simulink model "twoD_ground"  (R2022b)
settings: Solver=FixedStepAuto  StartTime=0.0  StopTime=1  FixedStep=10e-4  RelTol=1e-3
values from neighbouring files (symbols this model uses):
  bl = 0.1    [twoD.m]
  bw = 0.001    [twoD.m]
  g = 9.81    [twoD.m]
  I = m*(e^2 + n^2)/12    (= 0.001875)    [twoD.m]
  k0 = 1000    [twoD.m]
  Kf = acker(Af,Bf,Poles)    [twoD.m]
  l0 = 0.3    [twoD.m]
  m = 0.5    [twoD.m]
  Nf = rscale(Gp,Kf)    [twoD.m]
  Ng = rscale(sys,Kg)    [twoD.m]
undefined symbols (not defined in the file or in its folder): Kg
libraries: simulink x2
settings Model: Creator=phattanarat  LastModifiedBy=phattanarat

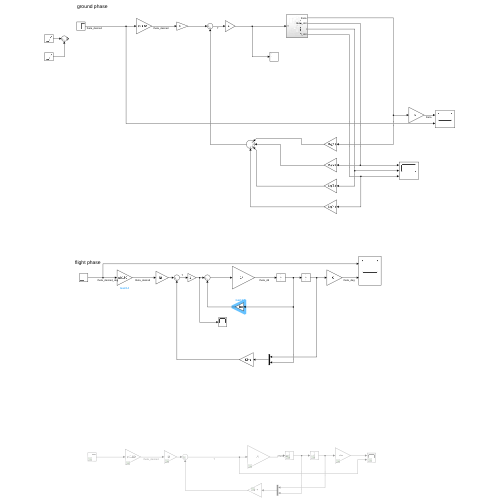
[thumbnail: Simulink's stored preview of the top-level diagram]
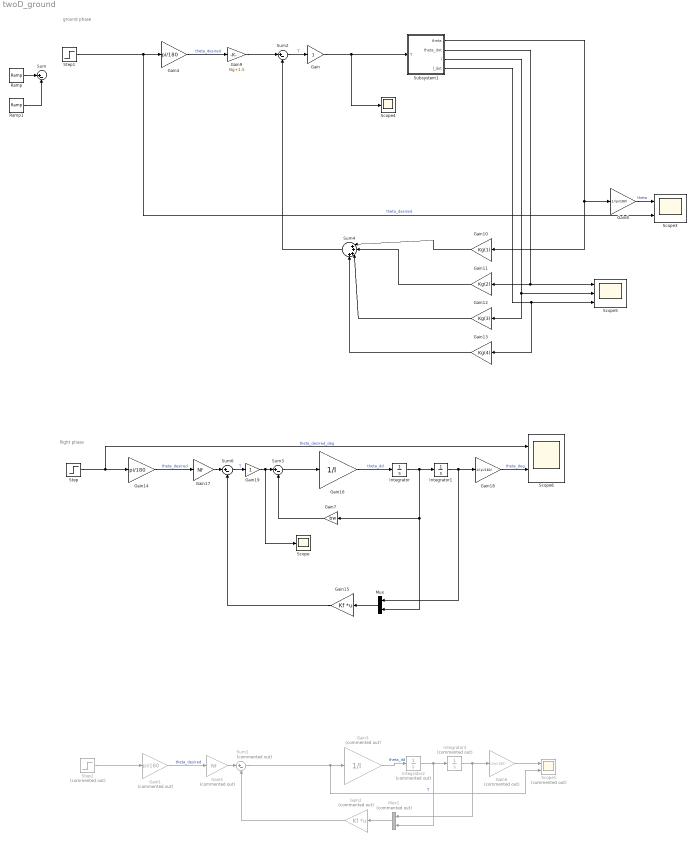
== system twoD_ground ==
  note: ground phase
  note: flight phase
  Gain : Gain
  Gain1 : Gain  Commented=on  Gain=pi/180
  Gain10 : Gain  Gain=Kg(1)
  Gain11 : Gain  Gain=Kg(2)
  Gain12 : Gain  Gain=Kg(3)
  Gain13 : Gain  Gain=Kg(4)
  Gain14 : Gain  Gain=pi/180
  Gain15 : Gain  Gain=Kf  Multiplication=Matrix(K*u)
  Gain16 : Gain  Gain=1/I
  Gain17 : Gain  Gain=Nf
  Gain18 : Gain  Gain=1/(pi/180)
  Gain19 : Gain
  Gain2 : Gain  Commented=on  Gain=Kf  Multiplication=Matrix(K*u)
  Gain3 : Gain  Commented=on  Gain=1/I
  Gain4 : Gain  Gain=pi/180
  Gain5 : Gain  Commented=on  Gain=Nf
  Gain6 : Gain  Commented=on  Gain=1/(pi/180)
  Gain7 : Gain  Gain=bw
  Gain8 : Gain  Gain=1/(pi/180)
  Gain9 : Gain  Gain=Ng+1.5
  Integrator : Integrator
  Integrator1 : Integrator  InitialCondition=93*pi/180
  Integrator2 : Integrator  Commented=on  InitialCondition=0.1
  Integrator3 : Integrator  Commented=on  InitialCondition=93*pi/180
  Mux : Mux  Inputs=2
  Mux1 : Mux  Commented=on  Inputs=2
  Ramp : simulink/Sources/Ramp  slope=40  start=0  InitialOutput=87
  Ramp1 : simulink/Sources/Ramp  slope=40  start=0.3  InitialOutput=0
  Scope : Scope
  Scope1 : Scope  Commented=on  NumInputPorts=2
  Scope3 : Scope  NumInputPorts=2
  Scope4 : Scope
  Scope5 : Scope  NumInputPorts=3
  Scope6 : Scope  NumInputPorts=2
  Step : Step  Time=0  After=90  SampleTime=0
  Step1 : Step  Time=0  After=93  SampleTime=0
  Step2 : Step  Commented=on  Time=0  After=87  SampleTime=0
  Subsystem1 : Subsystem
  Sum{,2..3,6} (4 alike) : Sum  Inputs=|+-
  Sum1 : Sum  Commented=on  Inputs=|+-
  Sum4 : Sum  Inputs=|++++
  wires:
  Subsystem1/2(theta_dot) -> Gain11/1, Scope5/1
  Gain9/1 -> Sum2/1
  Gain8/1 -> Scope3/1  "theta"
  Gain4/1 -> Gain9/1  "theta_desired"
  Sum2/1 -> Gain/1  "T"
  Step1/1 -> Scope3/2, Gain4/1  "theta_desired"
  Sum4/1 -> Sum2/2
  Subsystem1/1(theta) -> Gain10/1, Gain8/1
  Subsystem1/3(l) -> Gain12/1, Scope5/2
  Subsystem1/4(l_dot) -> Gain13/1, Scope5/3
  Gain10/1 -> Sum4/1
  Gain11/1 -> Sum4/2
  Gain14/1 -> Gain17/1  "theta_desired"
  Sum6/1 -> Gain19/1  "T"
  Integrator/1 -> Gain7/1, Mux/2, Integrator1/1
  Gain16/1 -> Integrator/1  "theta_dd"
  Integrator1/1 -> Mux/1, Gain18/1
  Mux/1 -> Gain15/1
  Gain15/1 -> Sum6/2
  Gain17/1 -> Sum6/1
  Gain18/1 -> Scope6/2  "theta_deg"
  Step/1 -> Scope6/1, Gain14/1  "theta_desired_deg"
  Ramp/1 -> Sum/1
  Ramp1/1 -> Sum/2
  Gain/1 -> Scope4/1, Subsystem1/1(T)
  Gain3/1 -> Integrator2/1  "theta_dd"
  Gain5/1 -> Sum1/1
  Integrator3/1 -> Mux1/1, Gain6/1
  Gain2/1 -> Sum1/2
  Integrator2/1 -> Mux1/2, Integrator3/1
  Sum1/1 -> Gain3/1, Scope1/2  "T"
  Step2/1 -> Gain1/1
  Mux1/1 -> Gain2/1
  Gain1/1 -> Gain5/1  "theta_desired"
  Gain6/1 -> Scope1/1
  Sum3/1 -> Gain16/1
  Gain7/1 -> Sum3/2
  Gain19/1 -> Scope/1, Sum3/1
  Gain12/1 -> Sum4/3
  Gain13/1 -> Sum4/4

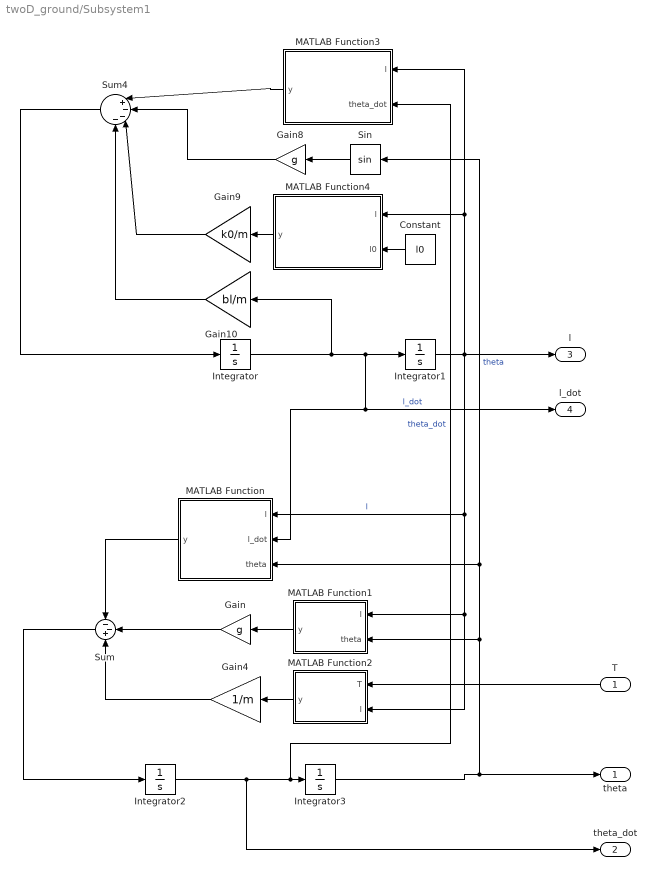
== system twoD_ground/Subsystem1 ==
  T : Inport
  Constant : Constant  Value=l0
  Gain : Gain  Gain=g
  Gain10 : Gain  Gain=bl/m
  Gain4 : Gain  Gain=1/m
  Gain8 : Gain  Gain=g
  Gain9 : Gain  Gain=k0/m
  Integrator : Integrator  InitialCondition=0.1
  Integrator1 : Integrator  InitialCondition=l0
  Integrator2 : Integrator
  Integrator3 : Integrator  InitialCondition=90*pi/180
  MATLAB Function : MATLAB Function  TreatAsAtomicUnit=on
  MATLAB Function1 : MATLAB Function  TreatAsAtomicUnit=on
  MATLAB Function2 : MATLAB Function  TreatAsAtomicUnit=on
  MATLAB Function3 : MATLAB Function  TreatAsAtomicUnit=on
  MATLAB Function4 : MATLAB Function  TreatAsAtomicUnit=on
  Sin : Trigonometry
  Sum : Sum  Inputs=--+
  Sum4 : Sum  Inputs=|+---
  theta : Outport
  theta_dot : Outport  Port=2
  l : Outport  Port=3
  l_dot : Outport  Port=4
  wires:
  MATLAB Function4/1(y) -> Gain9/1
  MATLAB Function2/1(y) -> Gain4/1
  MATLAB Function1/1(y) -> Gain/1
  Integrator1/1 -> MATLAB Function2/2(l), MATLAB Function1/1(l), MATLAB Function/1(l), l/1, MATLAB Function4/1(l), MATLAB Function3/1(l)  "l"
  Integrator2/1 -> theta_dot/1, MATLAB Function3/2(theta_dot), Integrator3/1  "theta_dot"
  Sin/1 -> Gain8/1
  Integrator/1 -> Gain10/1, l_dot/1, MATLAB Function/2(l_dot), Integrator1/1  "l_dot"
  Integrator3/1 -> theta/1, MATLAB Function1/2(theta), MATLAB Function/3(theta), Sin/1  "theta"
  Constant/1 -> MATLAB Function4/2(l0)
  Gain/1 -> Sum/2
  Sum/1 -> Integrator2/1
  MATLAB Function/1(y) -> Sum/1
  Gain4/1 -> Sum/3
  T/1 -> MATLAB Function2/1(T)
  Sum4/1 -> Integrator/1
  MATLAB Function3/1(y) -> Sum4/1
  Gain8/1 -> Sum4/2
  Gain9/1 -> Sum4/3
  Gain10/1 -> Sum4/4

== matlab function twoD_ground/Subsystem1/MATLAB Function1 ==
  data: l input; y output; theta input
function y = fcn(l,theta)

y = cos(theta)/l;

== matlab function twoD_ground/Subsystem1/MATLAB Function2 ==
  data: T input; l input; y output
function y = fcn(T,l)

y = T/l^2;

== matlab function twoD_ground/Subsystem1/MATLAB Function3 ==
  data: l input; y output; theta_dot input
function y = fcn(l,theta_dot)

y = l*theta_dot^2;

== matlab function twoD_ground/Subsystem1/MATLAB Function4 ==
  data: l input; y output; l0 input
function y = fcn(l,l0)

y = l-l0;

== matlab function twoD_ground/Subsystem1/MATLAB Function ==
  data: l input; l_dot input; y output; theta input
function y = fcn(l,l_dot,theta)

y = 2*l_dot*theta/l;
